simulink model "lib_nrhdlSignalDetection"  (R2023b)
settings: Solver=FixedStepDiscrete  StartTime=0.0  StopTime=sl_in.stopTime  RelTol=1e-3
undefined symbols (not defined in the file): sl_in
libraries: hdlsllib x5, simulink x4, dsphdlfiltering2 x4, dspsrcs4 x3, whdlmod x1
settings Model: DataTypeOverride=Off  SimulationMode=accelerator  Creator=The MathWorks, Inc.  LastModifiedBy=The MathWorks, Inc.
settings OptimizationCC: BlockReduction=off  ConditionallyExecuteInputs=off  DefaultParameterBehavior=Inlined  InheritOutputTypeSmallerThanSingle=on  ReuseModelBlockBuffer=off
settings DebuggingCC: AlgebraicLoopMsg=error  SingleTaskRateTransMsg=error  SubsystemReferenceDiagnosticForUnitTest=warning
settings HardwareCC: ProdBitPerPointer=32  ProdBitPerSizeT=32  ProdBitPerPtrDiffT=32  ProdLargestAtomicFloat=None  ProdIntDivRoundTo=Undefined  ProdEndianess=Unspecified  ProdWordSize=32  ProdHWDeviceType=ASIC/FPGA->ASIC/FPGA  TargetBitPerLong=64  TargetBitPerPointer=64  TargetBitPerSizeT=64  TargetBitPerPtrDiffT=64  TargetLongLongMode=on  TargetIntDivRoundTo=Zero  TargetEndianess=LittleEndian  TargetWordSize=64  TargetHWDeviceType=Custom Processor->MATLAB Host Computer  ProdEqTarget=off

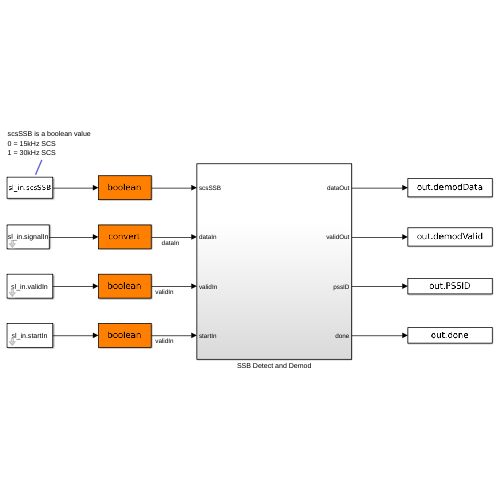
[thumbnail: Simulink's stored preview of the top-level diagram]
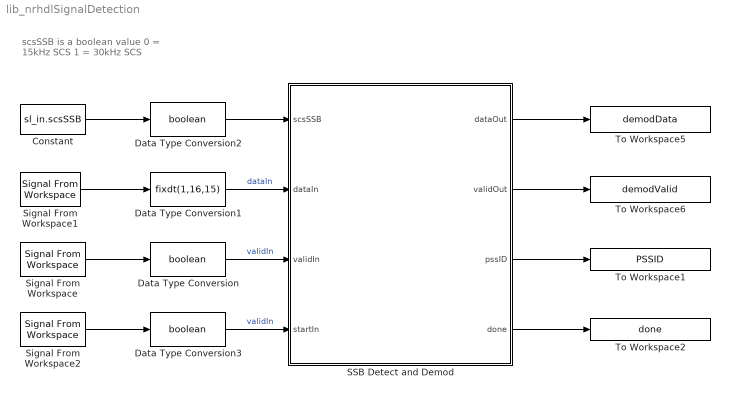
== system lib_nrhdlSignalDetection ==
  note: scsSSB is a boolean value
      | 0 = 15kHz SCS
      | 1 = 30kHz SCS
  Constant : Constant  Value=sl_in.scsSSB  SampleTime=sl_in.sampleTime
  Data Type Conversion : DataTypeConversion  OutDataTypeStr=boolean  SaturateOnIntegerOverflow=off  RndMeth=Floor
  Data Type Conversion1 : DataTypeConversion  OutDataTypeStr=fixdt(1,16,15)  RndMeth=Round  SaturateOnIntegerOverflow=off
  Data Type Conversion2 : DataTypeConversion  OutDataTypeStr=boolean  SaturateOnIntegerOverflow=off  RndMeth=Floor
  Data Type Conversion3 : DataTypeConversion  OutDataTypeStr=boolean  SaturateOnIntegerOverflow=off  RndMeth=Floor
  SSB Detect and Demod : Subsystem
  Signal From Workspace : dspsrcs4/Signal From Workspace  X=sl_in.validIn  Ts=sl_in.sampleTime  nsamps=1  OutputAfterFinalValue=Setting to zero  ignoreOrWarnInputAndFrameLengths=off  OutputFrames=off
  Signal From Workspace1 : dspsrcs4/Signal From Workspace  X=sl_in.signalIn  Ts=sl_in.sampleTime  nsamps=1  OutputAfterFinalValue=Setting to zero  ignoreOrWarnInputAndFrameLengths=off  OutputFrames=off
  Signal From Workspace2 : dspsrcs4/Signal From Workspace  X=sl_in.startIn  Ts=sl_in.sampleTime  nsamps=1  OutputAfterFinalValue=Setting to zero  ignoreOrWarnInputAndFrameLengths=off  OutputFrames=off
  To Workspace1 : ToWorkspace  VariableName=PSSID  SampleTime=-1
      settings: Save2DSignal=2-D array (concatenate along first dimension)
  To Workspace2 : ToWorkspace  VariableName=done  SampleTime=-1
      settings: Save2DSignal=2-D array (concatenate along first dimension)
  To Workspace5 : ToWorkspace  VariableName=demodData  SampleTime=-1
      settings: Save2DSignal=2-D array (concatenate along first dimension)
  To Workspace6 : ToWorkspace  VariableName=demodValid  SampleTime=-1
      settings: Save2DSignal=2-D array (concatenate along first dimension)
  wires:
  Signal From Workspace1/1 -> Data Type Conversion1/1
  Signal From Workspace/1 -> Data Type Conversion/1
  Data Type Conversion/1 -> SSB Detect and Demod/3(validIn)  "validIn"
  SSB Detect and Demod/1(dataOut) -> To Workspace5/1
  SSB Detect and Demod/2(validOut) -> To Workspace6/1
  Data Type Conversion1/1 -> SSB Detect and Demod/2(dataIn)  "dataIn"
  Constant/1 -> Data Type Conversion2/1
  SSB Detect and Demod/3(pssID) -> To Workspace1/1
  Data Type Conversion2/1 -> SSB Detect and Demod/1(scsSSB)
  Signal From Workspace2/1 -> Data Type Conversion3/1
  Data Type Conversion3/1 -> SSB Detect and Demod/4(startIn)  "validIn"
  SSB Detect and Demod/4(done) -> To Workspace2/1

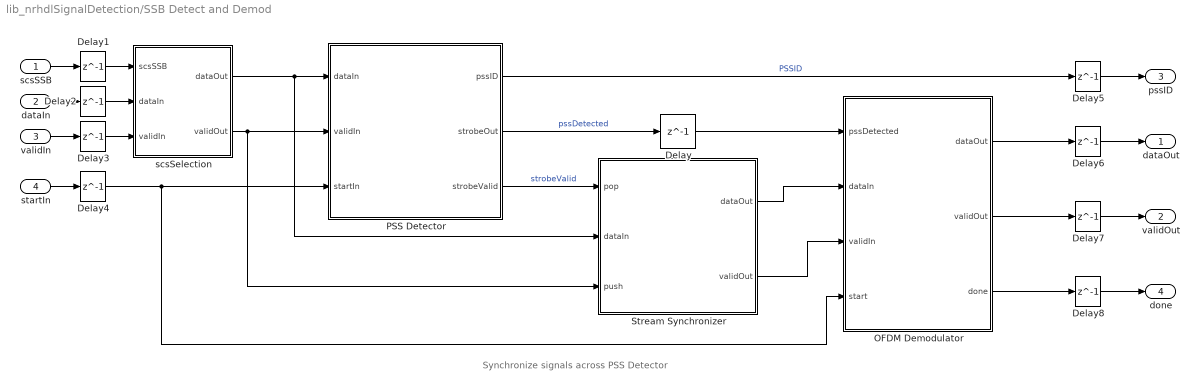
== system lib_nrhdlSignalDetection/SSB Detect and Demod ==
  note: Synchronize signals across PSS Detector
  scsSSB : Inport
  dataIn : Inport  Port=2
  validIn : Inport  Port=3
  startIn : Inport  Port=4
  Delay{,1..8} (9 alike) : Delay  DelayLength=1
  OFDM Demodulator : Subsystem
  PSS Detector : Subsystem
  Stream Synchronizer : Subsystem  mask{depth=512}
  scsSelection : Subsystem
  dataOut : Outport
  validOut : Outport  Port=2
  pssID : Outport  Port=3
  done : Outport  Port=4
  wires:
  OFDM Demodulator/1(dataOut) -> Delay6/1
  OFDM Demodulator/2(validOut) -> Delay7/1
  Stream Synchronizer/1(dataOut) -> OFDM Demodulator/2(dataIn)
  Stream Synchronizer/2(validOut) -> OFDM Demodulator/3(validIn)
  scsSelection/2(validOut) -> Stream Synchronizer/3(push), PSS Detector/2(validIn)
  PSS Detector/3(strobeValid) -> Stream Synchronizer/1(pop)  "strobeValid"
  scsSelection/1(dataOut) -> Stream Synchronizer/2(dataIn), PSS Detector/1(dataIn)
  PSS Detector/1(pssID) -> Delay5/1  "PSSID"
  scsSSB/1 -> Delay1/1
  validIn/1 -> Delay3/1
  dataIn/1 -> Delay2/1
  PSS Detector/2(strobeOut) -> Delay/1  "pssDetected"
  Delay/1 -> OFDM Demodulator/1(pssDetected)
  OFDM Demodulator/3(done) -> Delay8/1
  startIn/1 -> Delay4/1
  Delay1/1 -> scsSelection/1(scsSSB)
  Delay2/1 -> scsSelection/2(dataIn)
  Delay3/1 -> scsSelection/3(validIn)
  Delay4/1 -> OFDM Demodulator/4(start), PSS Detector/3(startIn)
  Delay5/1 -> pssID/1
  Delay6/1 -> dataOut/1
  Delay7/1 -> validOut/1
  Delay8/1 -> done/1

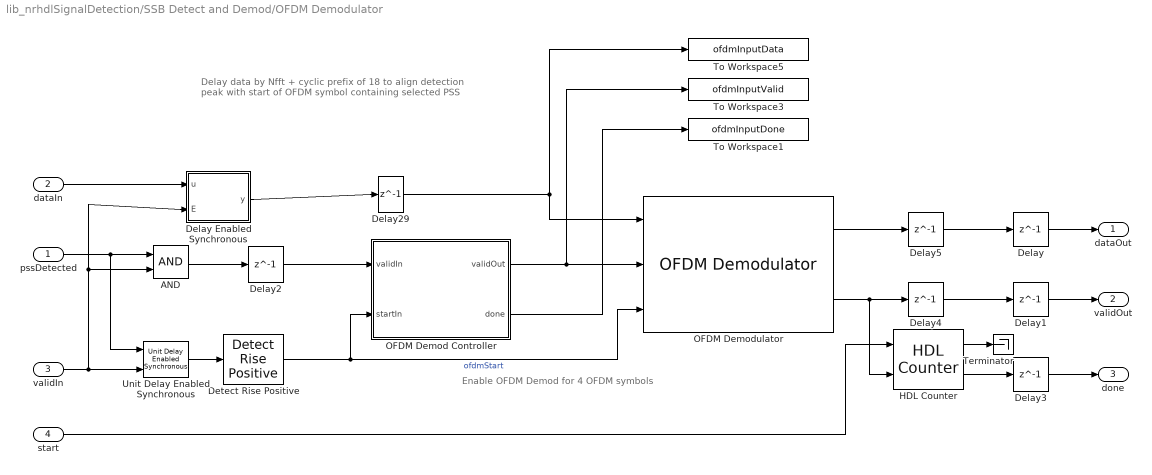
== system lib_nrhdlSignalDetection/SSB Detect and Demod/OFDM Demodulator ==
  note: Delay data by Nfft + cyclic prefix of 18 to align detection peak with start of OFDM symbol containing selected PSS
  note: Enable OFDM Demod for 4 OFDM symbols
  pssDetected : Inport
  dataIn : Inport  Port=2
  validIn : Inport  Port=3
  start : Inport  Port=4
  AND : Logic  AllPortsSameDT=off  OutDataTypeStr=boolean
  Delay{,1..5,29} (7 alike) : Delay  DelayLength=1
  Delay Enabled Synchronous : Subsystem  mask(Delay Enabled){DelayLength=256+18, InitialCondition=0.0}
      mask prompts: DelayLength "Simulink:blkprm_prompts:DelayBlkDelayLength"; InitialCondition "Simulink:blkprm_prompts:DelayBlkInitCond"
      mask help: Implements a delay with synchronous enable.
      mask TypeOptions DelayLength: Synchronous Delay/Delay/DelayLength
      mask TypeOptions InitialCondition: Synchronous Delay/Delay/InitialCondition
      mask DialogControl DelayLength Prompt: Delay length:
      mask DialogControl InitialCondition Prompt: Initial condition:
      mask Display:
      | port_label('input', 1, 'u');
      | port_label('input', 2, 'E');
      | text(0.45,0.45, 'Z');
      | DelayLengthStr = get_param(gcbh,'DelayLength');
      | try
      |     DelayLength = eval(DelayLengthStr);
      |     text(0.55,0.55, sprintf('-%d',DelayLength));
      | catch ME
      |     text(0.55,0.55, '-N');
      | end
  Detect Rise Positive : simulink/Logic and Bit Operations/Detect Rise Positive  vinit=0  OutDataTypeStr=boolean
  HDL Counter : hdlsllib/Sources/HDL Counter  CountType=Count limited  CountInit=0  CountStep=1  CountMax=960  CountFromType=Initial value  CountFrom=0  CountResetPort=on  CountLoadPort=off  CountEnbPort=on  CountDirPort=off  CountHitOutputPort=on  CountDataType=Unsigned  CountWordLen=12  CountFracLen=0  CountSampTime=1
  OFDM Demod Controller : MATLAB Function  TreatAsAtomicUnit=on
  OFDM Demodulator : whdlmod/OFDM Demodulator  OFDMParamsSource=Property  MaxFFTLength=256  FFTLength=256  CPLength=18  NumLGsC=8  NumRGsC=8  CPFraction=on  CPFractionSource=Property  CPFractionValue=0.5  removeDCSubcarriers=off  enableResetInputPort=on  Normalize=off  RoundingMethod=Round  SimulateUsing=Code generation
  Terminator : Terminator
  To Workspace1 : ToWorkspace  VariableName=ofdmInputDone  SampleTime=-1
      settings: Save2DSignal=2-D array (concatenate along first dimension)
  To Workspace3 : ToWorkspace  VariableName=ofdmInputValid  SampleTime=-1
      settings: Save2DSignal=2-D array (concatenate along first dimension)
  To Workspace5 : ToWorkspace  VariableName=ofdmInputData  SampleTime=-1
      settings: Save2DSignal=2-D array (concatenate along first dimension)
  Unit Delay Enabled Synchronous : hdlsllib/Discrete/Unit Delay Enabled Synchronous  InitialCondition=0.0  SampleTime=-1
  dataOut : Outport
  validOut : Outport  Port=2
  done : Outport  Port=3
  wires:
  AND/1 -> Delay2/1
  pssDetected/1 -> Unit Delay Enabled Synchronous/1, AND/1
  Unit Delay Enabled Synchronous/1 -> Detect Rise Positive/1
  dataIn/1 -> Delay Enabled Synchronous/1(u)
  Delay Enabled Synchronous/1(y) -> Delay29/1
  Delay29/1 -> OFDM Demodulator/1, To Workspace5/1
  Delay2/1 -> OFDM Demod Controller/1(validIn)
  Detect Rise Positive/1 -> OFDM Demodulator/3, OFDM Demod Controller/2(startIn)  "ofdmStart"
  OFDM Demod Controller/1(validOut) -> OFDM Demodulator/2, To Workspace3/1
  OFDM Demod Controller/2(done) -> To Workspace1/1
  HDL Counter/2 -> Delay3/1
  validIn/1 -> Delay Enabled Synchronous/2(E), AND/2, Unit Delay Enabled Synchronous/2
  HDL Counter/1 -> Terminator/1
  Delay/1 -> dataOut/1
  Delay1/1 -> validOut/1
  Delay3/1 -> done/1
  start/1 -> HDL Counter/1
  OFDM Demodulator/2 -> Delay4/1, HDL Counter/2
  OFDM Demodulator/1 -> Delay5/1
  Delay5/1 -> Delay/1
  Delay4/1 -> Delay1/1

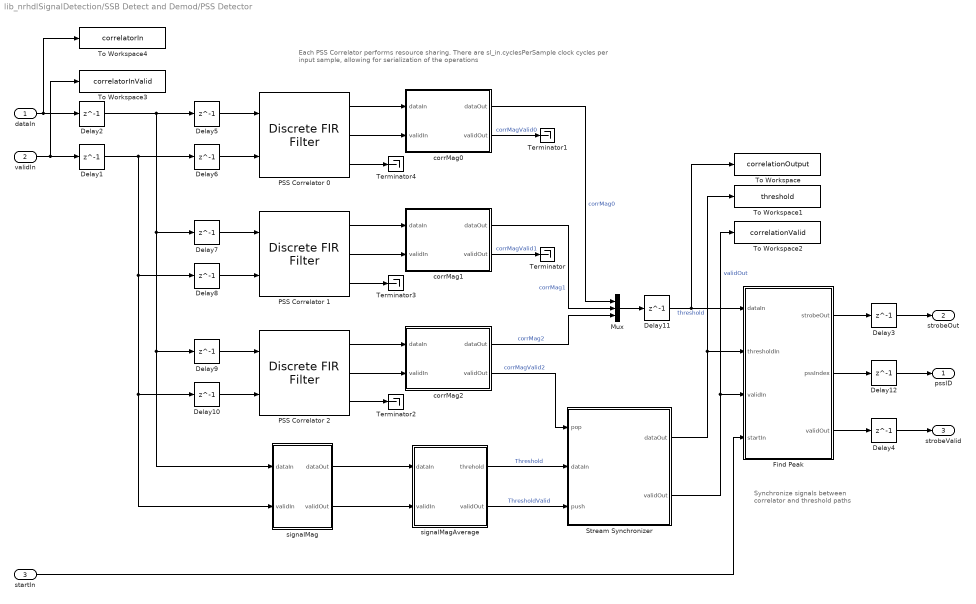
== system lib_nrhdlSignalDetection/SSB Detect and Demod/PSS Detector ==
  note: Each PSS Correlator performs resource sharing. There are sl_in.cyclesPerSample clock cycles per input sample, allowing for serialization of the operations
  note: Synchronize signals between correlator and threshold paths
  dataIn : Inport
  validIn : Inport  Port=2
  startIn : Inport  Port=3
  Delay{1..12} (12 alike) : Delay  DelayLength=1
  Find Peak : Subsystem
  Mux : Mux  Inputs=3
  PSS Correlator 0 : dsphdlfiltering2/Discrete FIR Filter  NumeratorSource=Property  Numerator=sl_in.pssCorrelationCoeffs(:,1).'  NumeratorPrototype=[]  FilterStructure=Partly serial systolic  SerializationOption=Minimum number of cycles between valid input samples  NumCycles=sl_in.cyclesPerSample  NumberOfMultipliers=2  SimulateUsing=Code generation  roundingMode=Floor  overflowMode=off  CoefficientsDataTypeStr=fixdt(1,8,10)  OutputDataTypeStr=fixdt(1,18,13)  ResetInputPort=off  HDLGlobalReset=off  CoeffMultiplier=Multiplier  UseMultForPow2Coeff=on
  PSS Correlator 1 : dsphdlfiltering2/Discrete FIR Filter  NumeratorSource=Property  Numerator=sl_in.pssCorrelationCoeffs(:,2).'  NumeratorPrototype=[]  FilterStructure=Partly serial systolic  SerializationOption=Minimum number of cycles between valid input samples  NumCycles=sl_in.cyclesPerSample  NumberOfMultipliers=2  SimulateUsing=Code generation  roundingMode=Floor  overflowMode=off  CoefficientsDataTypeStr=fixdt(1,8,10)  OutputDataTypeStr=fixdt(1,18,13)  ResetInputPort=off  HDLGlobalReset=off  CoeffMultiplier=Multiplier  UseMultForPow2Coeff=on
  PSS Correlator 2 : dsphdlfiltering2/Discrete FIR Filter  NumeratorSource=Property  Numerator=sl_in.pssCorrelationCoeffs(:,3).'  NumeratorPrototype=[]  FilterStructure=Partly serial systolic  SerializationOption=Minimum number of cycles between valid input samples  NumCycles=sl_in.cyclesPerSample  NumberOfMultipliers=2  SimulateUsing=Code generation  roundingMode=Floor  overflowMode=off  CoefficientsDataTypeStr=fixdt(1,8,10)  OutputDataTypeStr=fixdt(1,18,13)  ResetInputPort=off  HDLGlobalReset=off  CoeffMultiplier=Multiplier  UseMultForPow2Coeff=on
  Stream Synchronizer : Subsystem  mask{depth=512}
  Terminator{,1..4} (5 alike) : Terminator
  To Workspace : ToWorkspace  VariableName=correlationOutput  SampleTime=-1
      settings: Save2DSignal=2-D array (concatenate along first dimension)
  To Workspace1 : ToWorkspace  VariableName=threshold  SampleTime=-1
      settings: Save2DSignal=2-D array (concatenate along first dimension)
  To Workspace2 : ToWorkspace  VariableName=correlationValid  SampleTime=-1
      settings: Save2DSignal=2-D array (concatenate along first dimension)
  To Workspace3 : ToWorkspace  VariableName=correlatorInValid  SampleTime=-1
      settings: Save2DSignal=2-D array (concatenate along first dimension)
  To Workspace4 : ToWorkspace  VariableName=correlatorIn  SampleTime=-1
      settings: Save2DSignal=2-D array (concatenate along first dimension)
  corrMag0 : Subsystem
  corrMag1 : Subsystem
  corrMag2 : Subsystem
  signalMag : Subsystem
  signalMagAverage : Subsystem
  pssID : Outport
  strobeOut : Outport  Port=2
  strobeValid : Outport  Port=3
  wires:
  Stream Synchronizer/2(validOut) -> To Workspace2/1, Find Peak/3(validIn)  "validOut"
  Stream Synchronizer/1(dataOut) -> To Workspace1/1, Find Peak/2(thresholdIn)  "threshold"
  signalMagAverage/2(validOut) -> Stream Synchronizer/3(push)  "ThresholdValid"
  signalMagAverage/1(threhold) -> Stream Synchronizer/2(dataIn)  "Threshold"
  signalMag/2(validOut) -> signalMagAverage/2(validIn)
  signalMag/1(dataOut) -> signalMagAverage/1(dataIn)
  Delay4/1 -> strobeValid/1
  Find Peak/1(strobeOut) -> Delay3/1
  corrMag2/2(validOut) -> Stream Synchronizer/1(pop)  "corrMagValid2"
  Find Peak/3(validOut) -> Delay4/1
  validIn/1 -> To Workspace3/1, Delay1/1
  PSS Correlator 2/1 -> corrMag2/1(dataIn)
  PSS Correlator 2/2 -> corrMag2/2(validIn)
  dataIn/1 -> To Workspace4/1, Delay2/1
  PSS Correlator 1/2 -> corrMag1/2(validIn)
  PSS Correlator 1/1 -> corrMag1/1(dataIn)
  PSS Correlator 0/1 -> corrMag0/1(dataIn)
  PSS Correlator 0/2 -> corrMag0/2(validIn)
  corrMag1/2(validOut) -> Terminator/1  "corrMagValid1"
  corrMag0/2(validOut) -> Terminator1/1  "corrMagValid0"
  Delay5/1 -> PSS Correlator 0/1
  Delay6/1 -> PSS Correlator 0/2
  Delay8/1 -> PSS Correlator 1/2
  Delay7/1 -> PSS Correlator 1/1
  Delay9/1 -> PSS Correlator 2/1
  Delay1/1 -> signalMag/2(validIn), Delay10/1, Delay8/1, Delay6/1
  Delay10/1 -> PSS Correlator 2/2
  Delay2/1 -> Delay9/1, signalMag/1(dataIn), Delay7/1, Delay5/1
  PSS Correlator 2/3 -> Terminator2/1
  PSS Correlator 1/3 -> Terminator3/1
  PSS Correlator 0/3 -> Terminator4/1
  corrMag0/1(dataOut) -> Mux/1  "corrMag0"
  corrMag1/1(dataOut) -> Mux/2  "corrMag1"
  corrMag2/1(dataOut) -> Mux/3  "corrMag2"
  Delay3/1 -> strobeOut/1
  Find Peak/2(pssIndex) -> Delay12/1
  Delay12/1 -> pssID/1
  Mux/1 -> Delay11/1
  Delay11/1 -> To Workspace/1, Find Peak/1(dataIn)
  startIn/1 -> Find Peak/4(startIn)

== system lib_nrhdlSignalDetection/SSB Detect and Demod/Stream Synchronizer ==
  pop : Inport
  dataIn : Inport  Port=2
  push : Inport  Port=3
  MATLAB Function : MATLAB Function  InitFcn=Simulink.suppressDiagnostic(gcb, 'Stateflow:Runtime:DataOverflowErrorMSLD');  TreatAsAtomicUnit=on
  Simple Dual Port RAM System : hdlsllib/HDL RAMs/Simple Dual Port RAM System  RAMType=Simple dual port  AsyncRead=off  WriteOutputValue=New data  RAMInitialValue=0  allowBusInputs=off  WritesHaveOutput=on  NumReads=0  NumWrites=1  SimulateUsing=Code generation
  dataOut : Outport
  validOut : Outport  Port=2
  wires:
  Simple Dual Port RAM System/1 -> dataOut/1
  dataIn/1 -> Simple Dual Port RAM System/1
  pop/1 -> MATLAB Function/1(pop)
  push/1 -> MATLAB Function/2(push)
  MATLAB Function/4(validOut) -> validOut/1
  MATLAB Function/1(wrAddr) -> Simple Dual Port RAM System/2
  MATLAB Function/2(wrEn) -> Simple Dual Port RAM System/3
  MATLAB Function/3(rdAddr) -> Simple Dual Port RAM System/4

== system lib_nrhdlSignalDetection/SSB Detect and Demod/scsSelection ==
  note: 0 = 15kHz SCS
      | 1 = 30kHz SCS
  note: Decimate to 15KHz SCS rate
  note: convert to sfix16_15 to match filter input data type
  scsSSB : Inport
  dataIn : Inport  Port=2
  validIn : Inport  Port=3
  Data Type Conversion : DataTypeConversion  OutDataTypeStr=fixdt(1,16,15)  RndMeth=Round  SaturateOnIntegerOverflow=off
  FIR Decimator : dsphdlfiltering2/FIR Decimator  Numerator=sl_in.halfbandCoeffs  FilterStructure=Direct form systolic  DecimationFactor=2  NumCycles=sl_in.cyclesPerSample  SimulateUsing=Code generation  roundingMode=Round  overflowMode=off  CoefficientsDataTypeStr=fixdt(1,16,16)  ResetInputPort=off  HDLGlobalReset=off
  Multiport Switch : MultiPortSwitch  DataPortOrder=Zero-based contiguous  Inputs=2  zeroidx=on  SaturateOnIntegerOverflow=off  InputSameDT=off
  Multiport Switch1 : MultiPortSwitch  DataPortOrder=Zero-based contiguous  Inputs=2  zeroidx=on  SaturateOnIntegerOverflow=off  InputSameDT=off
  Transient Removal : MATLAB Function  TreatAsAtomicUnit=on  mask{TransientLength=sl_in.halfbandTransient}
      mask prompts: TransientLength "Transient length"
  dataOut : Outport
  validOut : Outport  Port=2
  wires:
  Multiport Switch/1 -> dataOut/1
  Multiport Switch1/1 -> validOut/1
  scsSSB/1 -> Multiport Switch1/1, Multiport Switch/1
  FIR Decimator/1 -> Data Type Conversion/1
  dataIn/1 -> Multiport Switch/3, FIR Decimator/1
  validIn/1 -> Multiport Switch1/3, FIR Decimator/2
  FIR Decimator/2 -> Transient Removal/2(validIn)
  Data Type Conversion/1 -> Transient Removal/1(dataIn)
  Transient Removal/1(dataOut) -> Multiport Switch/2
  Transient Removal/2(validOut) -> Multiport Switch1/2

== system lib_nrhdlSignalDetection/SSB Detect and Demod/OFDM Demodulator/Delay Enabled Synchronous ==
  u : Inport
  E : Inport  Port=2
  Synchronous Delay : Subsystem
  y : Outport
  wires:
  Synchronous Delay/1(y) -> y/1
  E/1 -> Synchronous Delay/2(E)
  u/1 -> Synchronous Delay/1(u)

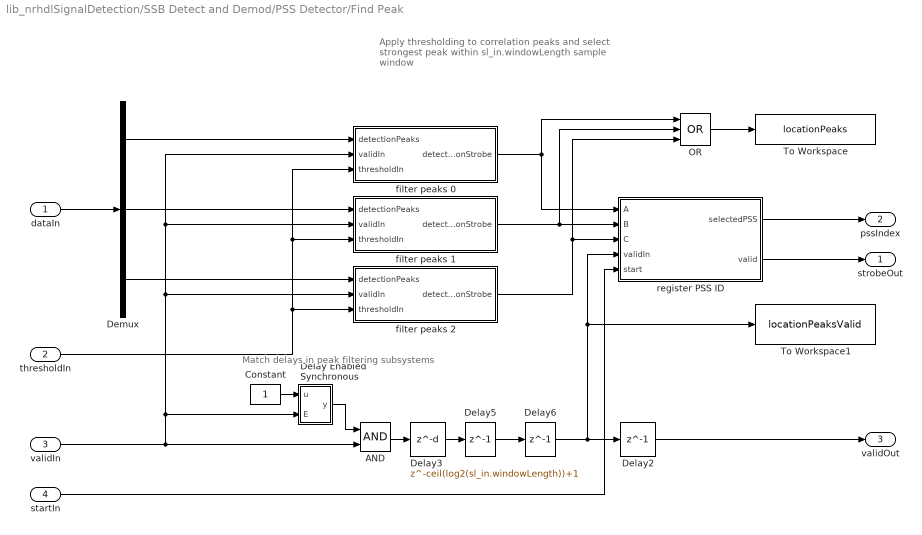
== system lib_nrhdlSignalDetection/SSB Detect and Demod/PSS Detector/Find Peak ==
  note: Match delays in peak filtering subsystems
  note: Apply thresholding to correlation peaks and select strongest peak within sl_in.windowLength sample window
  dataIn : Inport
  thresholdIn : Inport  Port=2
  validIn : Inport  Port=3
  startIn : Inport  Port=4
  AND : Logic  AllPortsSameDT=off  OutDataTypeStr=boolean
  Constant : Constant  OutDataTypeStr=boolean  SampleTime=-1
  Delay Enabled Synchronous : Subsystem  mask(Delay Enabled){DelayLength=ceil(sl_in.windowLength/2), InitialCondition=0.0}
      mask prompts: DelayLength "Simulink:blkprm_prompts:DelayBlkDelayLength"; InitialCondition "Simulink:blkprm_prompts:DelayBlkInitCond"
      mask help: Implements a delay with synchronous enable.
      mask TypeOptions DelayLength: Synchronous Delay/Delay/DelayLength
      mask TypeOptions InitialCondition: Synchronous Delay/Delay/InitialCondition
      mask DialogControl DelayLength Prompt: Delay length:
      mask DialogControl InitialCondition Prompt: Initial condition:
      mask Display:
      | port_label('input', 1, 'u');
      | port_label('input', 2, 'E');
      | text(0.45,0.45, 'Z');
      | DelayLengthStr = get_param(gcbh,'DelayLength');
      | try
      |     DelayLength = eval(DelayLengthStr);
      |     text(0.55,0.55, sprintf('-%d',DelayLength));
      | catch ME
      |     text(0.55,0.55, '-N');
      | end
  Delay2 : Delay  DelayLength=1
  Delay3 : Delay  DelayLength=ceil(log2(sl_in.windowLength))+1
  Delay5 : Delay  DelayLength=1
  Delay6 : Delay  DelayLength=1
  Demux : Demux  Outputs=3
  OR : Logic  Operator=OR  Inputs=3  AllPortsSameDT=off  OutDataTypeStr=boolean
  To Workspace : ToWorkspace  VariableName=locationPeaks  SampleTime=-1
      settings: Save2DSignal=2-D array (concatenate along first dimension)
  To Workspace1 : ToWorkspace  VariableName=locationPeaksValid  SampleTime=-1
      settings: Save2DSignal=2-D array (concatenate along first dimension)
  filter peaks 0 : Subsystem
  filter peaks 1 : Subsystem
  filter peaks 2 : Subsystem
  register PSS ID : MATLAB Function  TreatAsAtomicUnit=on
  strobeOut : Outport
  pssIndex : Outport  Port=2
  validOut : Outport  Port=3
  wires:
  Delay6/1 -> register PSS ID/4(validIn), To Workspace1/1, Delay2/1
  Delay5/1 -> Delay6/1
  validIn/1 -> AND/2, filter peaks 2/2(validIn), filter peaks 1/2(validIn), filter peaks 0/2(validIn), Delay Enabled Synchronous/2(E)
  dataIn/1 -> Demux/1
  register PSS ID/1(selectedPSS) -> pssIndex/1
  Demux/2 -> filter peaks 1/1(detectionPeaks)
  Demux/3 -> filter peaks 2/1(detectionPeaks)
  thresholdIn/1 -> filter peaks 2/3(thresholdIn), filter peaks 1/3(thresholdIn), filter peaks 0/3(thresholdIn)
  Demux/1 -> filter peaks 0/1(detectionPeaks)
  filter peaks 0/1(detectionStrobe) -> OR/1, register PSS ID/1(A)
  filter peaks 1/1(detectionStrobe) -> OR/2, register PSS ID/2(B)
  filter peaks 2/1(detectionStrobe) -> OR/3, register PSS ID/3(C)
  register PSS ID/2(valid) -> strobeOut/1
  Delay2/1 -> validOut/1
  OR/1 -> To Workspace/1
  Delay Enabled Synchronous/1(y) -> AND/1
  Constant/1 -> Delay Enabled Synchronous/1(u)
  AND/1 -> Delay3/1
  startIn/1 -> register PSS ID/5(start)
  Delay3/1 -> Delay5/1

== system lib_nrhdlSignalDetection/SSB Detect and Demod/PSS Detector/Stream Synchronizer ==
  pop : Inport
  dataIn : Inport  Port=2
  push : Inport  Port=3
  MATLAB Function : MATLAB Function  InitFcn=Simulink.suppressDiagnostic(gcb, 'Stateflow:Runtime:DataOverflowErrorMSLD');  TreatAsAtomicUnit=on
  Simple Dual Port RAM System : hdlsllib/HDL RAMs/Simple Dual Port RAM System  RAMType=Simple dual port  AsyncRead=off  WriteOutputValue=New data  RAMInitialValue=0  allowBusInputs=off  WritesHaveOutput=on  NumReads=0  NumWrites=1  SimulateUsing=Code generation
  dataOut : Outport
  validOut : Outport  Port=2
  wires:
  Simple Dual Port RAM System/1 -> dataOut/1
  dataIn/1 -> Simple Dual Port RAM System/1
  pop/1 -> MATLAB Function/1(pop)
  push/1 -> MATLAB Function/2(push)
  MATLAB Function/4(validOut) -> validOut/1
  MATLAB Function/1(wrAddr) -> Simple Dual Port RAM System/2
  MATLAB Function/2(wrEn) -> Simple Dual Port RAM System/3
  MATLAB Function/3(rdAddr) -> Simple Dual Port RAM System/4

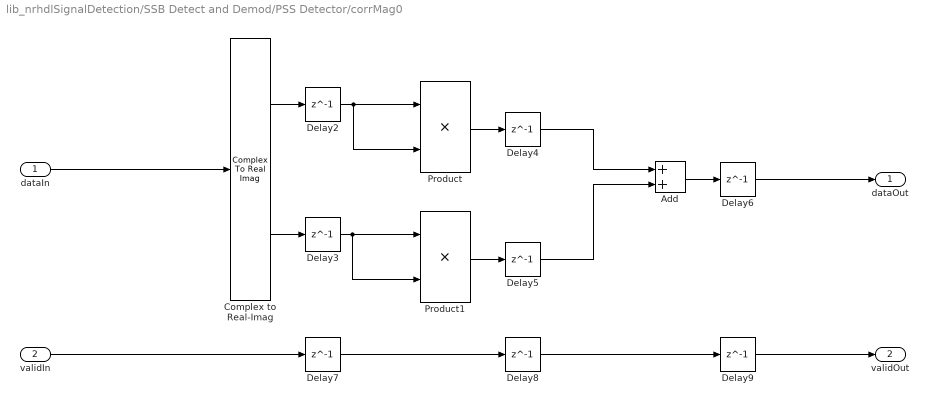
== system lib_nrhdlSignalDetection/SSB Detect and Demod/PSS Detector/corrMag0 ==
  dataIn : Inport
  validIn : Inport  Port=2
  Add : Sum  OutDataTypeStr=Inherit: Same as accumulator
  Complex to Real-Imag : ComplexToRealImag
  Delay{2..9} (8 alike) : Delay  DelayLength=1
  Product : Product
  Product1 : Product
  dataOut : Outport
  validOut : Outport  Port=2
  wires:
  validIn/1 -> Delay7/1
  dataIn/1 -> Complex to Real-Imag/1
  Product/1 -> Delay4/1
  Delay3/1 -> Product1/1, Product1/2
  Delay7/1 -> Delay8/1
  Delay5/1 -> Add/2
  Delay6/1 -> dataOut/1
  Product1/1 -> Delay5/1
  Delay9/1 -> validOut/1
  Delay4/1 -> Add/1
  Complex to Real-Imag/2 -> Delay3/1
  Delay8/1 -> Delay9/1
  Complex to Real-Imag/1 -> Delay2/1
  Add/1 -> Delay6/1
  Delay2/1 -> Product/1, Product/2

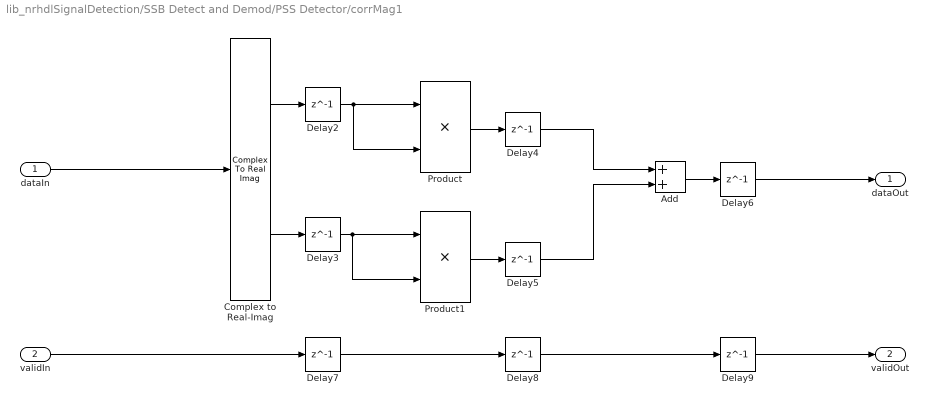
== system lib_nrhdlSignalDetection/SSB Detect and Demod/PSS Detector/corrMag1 ==
  dataIn : Inport
  validIn : Inport  Port=2
  Add : Sum  OutDataTypeStr=Inherit: Same as accumulator
  Complex to Real-Imag : ComplexToRealImag
  Delay{2..9} (8 alike) : Delay  DelayLength=1
  Product : Product
  Product1 : Product
  dataOut : Outport
  validOut : Outport  Port=2
  wires:
  Delay2/1 -> Product/2, Product/1
  Add/1 -> Delay6/1
  Complex to Real-Imag/1 -> Delay2/1
  Delay8/1 -> Delay9/1
  Complex to Real-Imag/2 -> Delay3/1
  Delay4/1 -> Add/1
  Delay9/1 -> validOut/1
  Product1/1 -> Delay5/1
  Delay6/1 -> dataOut/1
  Delay5/1 -> Add/2
  Delay7/1 -> Delay8/1
  Delay3/1 -> Product1/2, Product1/1
  Product/1 -> Delay4/1
  dataIn/1 -> Complex to Real-Imag/1
  validIn/1 -> Delay7/1

== system lib_nrhdlSignalDetection/SSB Detect and Demod/PSS Detector/corrMag2 ==
  dataIn : Inport
  validIn : Inport  Port=2
  Add : Sum  OutDataTypeStr=Inherit: Same as accumulator
  Complex to Real-Imag : ComplexToRealImag
  Delay{2..9} (8 alike) : Delay  DelayLength=1
  Product : Product
  Product1 : Product
  dataOut : Outport
  validOut : Outport  Port=2
  wires:
  validIn/1 -> Delay7/1
  dataIn/1 -> Complex to Real-Imag/1
  Product/1 -> Delay4/1
  Delay3/1 -> Product1/1, Product1/2
  Delay7/1 -> Delay8/1
  Delay5/1 -> Add/2
  Delay6/1 -> dataOut/1
  Product1/1 -> Delay5/1
  Delay9/1 -> validOut/1
  Delay4/1 -> Add/1
  Complex to Real-Imag/2 -> Delay3/1
  Delay8/1 -> Delay9/1
  Complex to Real-Imag/1 -> Delay2/1
  Add/1 -> Delay6/1
  Delay2/1 -> Product/1, Product/2

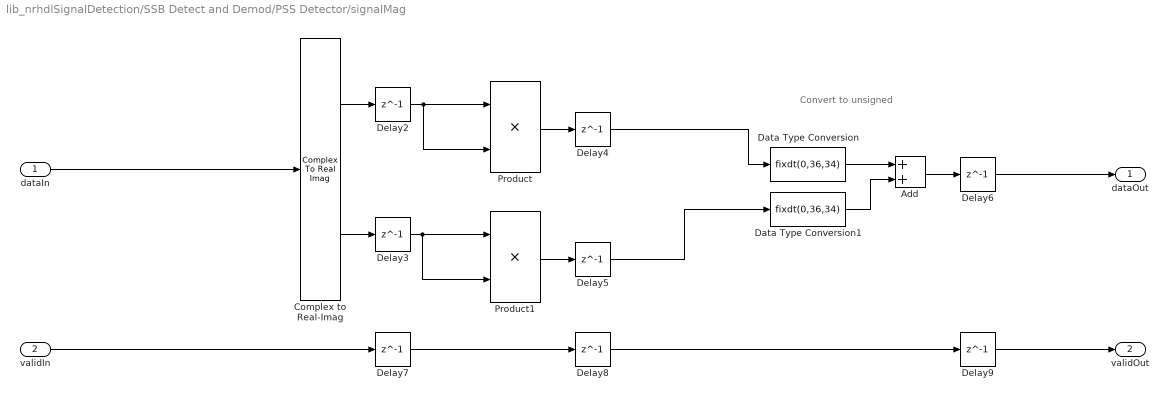
== system lib_nrhdlSignalDetection/SSB Detect and Demod/PSS Detector/signalMag ==
  note: Convert to unsigned
  dataIn : Inport
  validIn : Inport  Port=2
  Add : Sum
  Complex to Real-Imag : ComplexToRealImag
  Data Type Conversion : DataTypeConversion  OutDataTypeStr=fixdt(0,36,34)  SaturateOnIntegerOverflow=off  RndMeth=Floor
  Data Type Conversion1 : DataTypeConversion  OutDataTypeStr=fixdt(0,36,34)  SaturateOnIntegerOverflow=off  RndMeth=Floor
  Delay{2..9} (8 alike) : Delay  DelayLength=1
  Product : Product
  Product1 : Product
  dataOut : Outport
  validOut : Outport  Port=2
  wires:
  Data Type Conversion1/1 -> Add/2
  Data Type Conversion/1 -> Add/1
  Delay2/1 -> Product/2, Product/1
  Add/1 -> Delay6/1
  Complex to Real-Imag/1 -> Delay2/1
  Delay8/1 -> Delay9/1
  Complex to Real-Imag/2 -> Delay3/1
  Delay4/1 -> Data Type Conversion/1
  Delay9/1 -> validOut/1
  Product1/1 -> Delay5/1
  Delay6/1 -> dataOut/1
  Delay5/1 -> Data Type Conversion1/1
  Delay7/1 -> Delay8/1
  Delay3/1 -> Product1/2, Product1/1
  Product/1 -> Delay4/1
  dataIn/1 -> Complex to Real-Imag/1
  validIn/1 -> Delay7/1

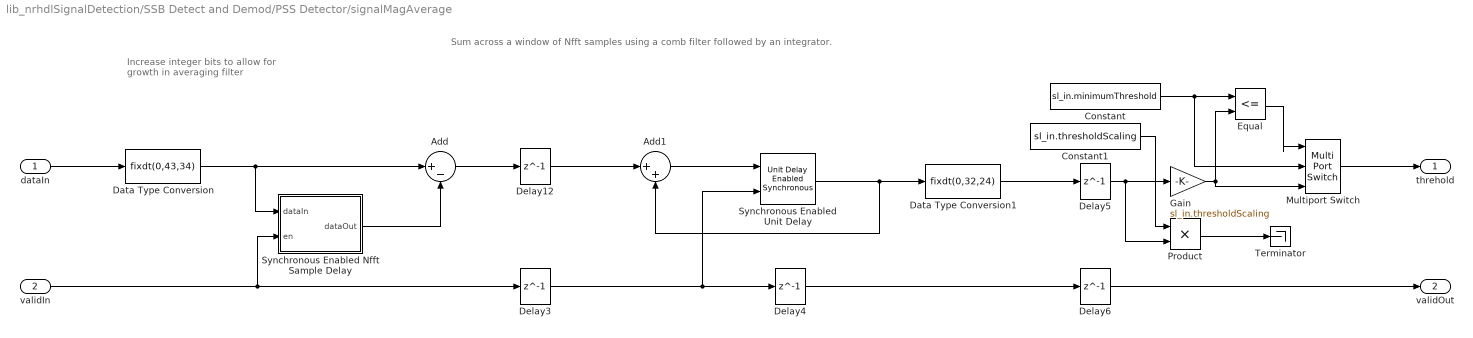
== system lib_nrhdlSignalDetection/SSB Detect and Demod/PSS Detector/signalMagAverage ==
  note: Increase integer bits to allow for growth in averaging filter
  note: Sum across a window of Nfft samples using a comb filter followed by an integrator.
  dataIn : Inport
  validIn : Inport  Port=2
  Add : Sum  Inputs=|+-  OutDataTypeStr=Inherit: Same as accumulator
  Add1 : Sum  Inputs=|++  OutDataTypeStr=Inherit: Same as accumulator
  Constant : Constant  Value=sl_in.minimumThreshold  SampleTime=-1
  Constant1 : Constant  Value=sl_in.thresholdScaling  SampleTime=-1
  Data Type Conversion : DataTypeConversion  OutDataTypeStr=fixdt(0,43,34)  SaturateOnIntegerOverflow=off  RndMeth=Floor
  Data Type Conversion1 : DataTypeConversion  OutDataTypeStr=fixdt(0,32,24)  SaturateOnIntegerOverflow=off  RndMeth=Floor
  Delay{3..6,12} (5 alike) : Delay  DelayLength=1  InitialCondition=0
  Equal : RelationalOperator  Operator=<=  OutDataTypeStr=boolean  RndMeth=Simplest  InputSameDT=off
  Gain : Gain  Gain=sl_in.thresholdScaling  ParamDataTypeStr=Inherit: Inherit from 'Gain'  OutDataTypeStr=Inherit: Same as input
  Multiport Switch : MultiPortSwitch  DataPortOrder=Zero-based contiguous  Inputs=2  zeroidx=on  SaturateOnIntegerOverflow=off  InputSameDT=off
  Product : Product
  "Synchronous Enabled Nfft Sample Delay " : Subsystem
  Synchronous Enabled Unit Delay : hdlsllib/Discrete/Unit Delay Enabled Synchronous  InitialCondition=0.0  SampleTime=-1
  Terminator : Terminator
  threhold : Outport  VectorParamsAs1DForOutWhenUnconnected=off
  validOut : Outport  Port=2  VectorParamsAs1DForOutWhenUnconnected=off
  wires:
  "Synchronous Enabled Nfft Sample Delay "/1(dataOut) -> Add/2
  Data Type Conversion1/1 -> Delay5/1
  Data Type Conversion/1 -> Add/1, "Synchronous Enabled Nfft Sample Delay "/1(dataIn)
  Delay6/1 -> validOut/1
  Delay5/1 -> Product/2, Gain/1
  Delay4/1 -> Delay6/1
  Delay3/1 -> Delay4/1, Synchronous Enabled Unit Delay/2
  Delay12/1 -> Add1/1
  validIn/1 -> Delay3/1, "Synchronous Enabled Nfft Sample Delay "/2(en)
  Add/1 -> Delay12/1
  Add1/1 -> Synchronous Enabled Unit Delay/1
  dataIn/1 -> Data Type Conversion/1
  Synchronous Enabled Unit Delay/1 -> Add1/2, Data Type Conversion1/1
  Equal/1 -> Multiport Switch/1
  Constant/1 -> Multiport Switch/2, Equal/1
  Gain/1 -> Equal/2, Multiport Switch/3
  Multiport Switch/1 -> threhold/1
  Constant1/1 -> Product/1
  Product/1 -> Terminator/1

== system lib_nrhdlSignalDetection/SSB Detect and Demod/OFDM Demodulator/Delay Enabled Synchronous/Synchronous Delay ==
  u : Inport
  E : Inport  Port=2
  Delay : Delay  DelayLength=DelayLength  InitialCondition=InitialCondition  ShowEnablePort=on
      settings: InputPortMap=u0,e6
  State Control : StateControl  StateControl=Synchronous
  y : Outport
  wires:
  u/1 -> Delay/1
  E/1 -> Delay/2
  Delay/1 -> y/1

== system lib_nrhdlSignalDetection/SSB Detect and Demod/PSS Detector/Find Peak/Delay Enabled Synchronous ==
  u : Inport
  E : Inport  Port=2
  Synchronous Delay : Subsystem
  y : Outport
  wires:
  Synchronous Delay/1(y) -> y/1
  E/1 -> Synchronous Delay/2(E)
  u/1 -> Synchronous Delay/1(u)

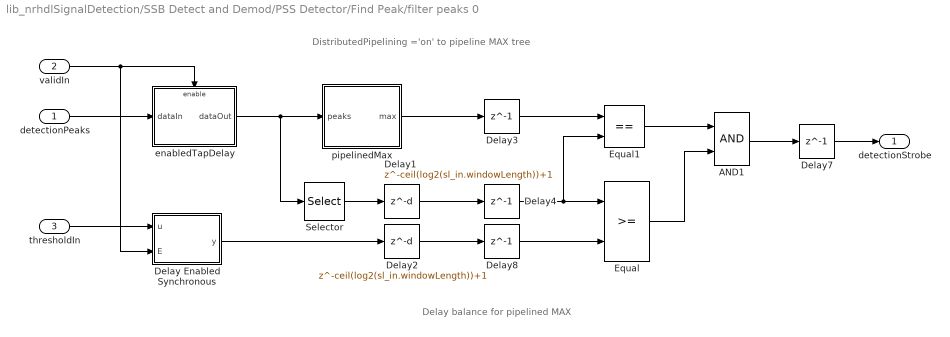
== system lib_nrhdlSignalDetection/SSB Detect and Demod/PSS Detector/Find Peak/filter peaks 0 ==
  note: Delay balance for pipelined MAX
  note: DistributedPipelining ='on' to pipeline MAX tree
  detectionPeaks : Inport
  validIn : Inport  Port=2
  thresholdIn : Inport  Port=3
  AND1 : Logic  AllPortsSameDT=off  OutDataTypeStr=boolean
  Delay Enabled Synchronous : Subsystem  mask(Delay Enabled){DelayLength=ceil(sl_in.windowLength/2), InitialCondition=0.0}
      mask prompts: DelayLength "Simulink:blkprm_prompts:DelayBlkDelayLength"; InitialCondition "Simulink:blkprm_prompts:DelayBlkInitCond"
      mask help: Implements a delay with synchronous enable.
      mask TypeOptions DelayLength: Synchronous Delay/Delay/DelayLength
      mask TypeOptions InitialCondition: Synchronous Delay/Delay/InitialCondition
      mask DialogControl DelayLength Prompt: Delay length:
      mask DialogControl InitialCondition Prompt: Initial condition:
      mask Display:
      | port_label('input', 1, 'u');
      | port_label('input', 2, 'E');
      | text(0.45,0.45, 'Z');
      | DelayLengthStr = get_param(gcbh,'DelayLength');
      | try
      |     DelayLength = eval(DelayLengthStr);
      |     text(0.55,0.55, sprintf('-%d',DelayLength));
      | catch ME
      |     text(0.55,0.55, '-N');
      | end
  Delay1 : Delay  DelayLength=ceil(log2(sl_in.windowLength))+1
  Delay2 : Delay  DelayLength=ceil(log2(sl_in.windowLength))+1
  Delay3 : Delay  DelayLength=1
  Delay4 : Delay  DelayLength=1
  Delay7 : Delay  DelayLength=1
  Delay8 : Delay  DelayLength=1  InitialCondition=1
  Equal : RelationalOperator  OutDataTypeStr=boolean  RndMeth=Simplest  InputSameDT=off
  Equal1 : RelationalOperator  Operator===  OutDataTypeStr=boolean  RndMeth=Simplest  InputSameDT=off
  Selector : Selector  InputPortWidth=sl_in.windowLength  IndexOptions=Index vector (dialog)  Indices=ceil(sl_in.windowLength/2)  OutputSizes=1
  enabledTapDelay : Subsystem
  pipelinedMax : Subsystem
  detectionStrobe : Outport
  wires:
  Equal1/1 -> AND1/1
  Delay4/1 -> Equal1/2, Equal/1
  Delay3/1 -> Equal1/1
  Equal/1 -> AND1/2
  AND1/1 -> Delay7/1
  Selector/1 -> Delay1/1
  Delay8/1 -> Equal/2
  Delay7/1 -> detectionStrobe/1
  thresholdIn/1 -> Delay Enabled Synchronous/1(u)
  validIn/1 -> Delay Enabled Synchronous/2(E), enabledTapDelay/Enable
  Delay Enabled Synchronous/1(y) -> Delay2/1
  enabledTapDelay/1(dataOut) -> Selector/1, pipelinedMax/1(peaks)
  detectionPeaks/1 -> enabledTapDelay/1(dataIn)
  pipelinedMax/1(max) -> Delay3/1
  Delay1/1 -> Delay4/1
  Delay2/1 -> Delay8/1

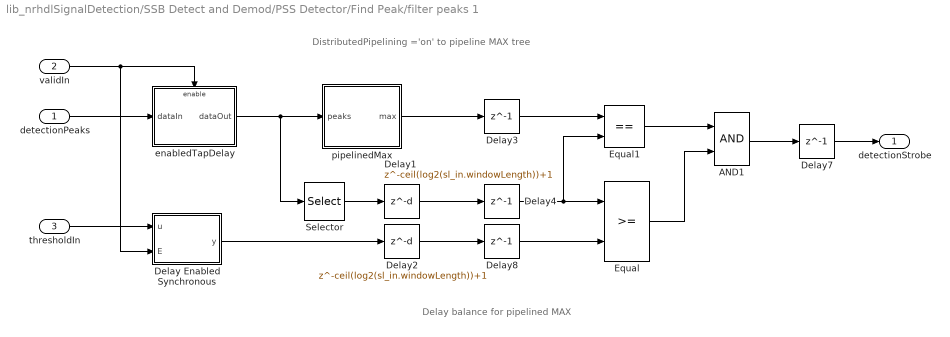
== system lib_nrhdlSignalDetection/SSB Detect and Demod/PSS Detector/Find Peak/filter peaks 1 ==
  note: DistributedPipelining ='on' to pipeline MAX tree
  note: Delay balance for pipelined MAX
  detectionPeaks : Inport
  validIn : Inport  Port=2
  thresholdIn : Inport  Port=3
  AND1 : Logic  AllPortsSameDT=off  OutDataTypeStr=boolean
  Delay Enabled Synchronous : Subsystem  mask(Delay Enabled){DelayLength=ceil(sl_in.windowLength/2), InitialCondition=0.0}
      mask prompts: DelayLength "Simulink:blkprm_prompts:DelayBlkDelayLength"; InitialCondition "Simulink:blkprm_prompts:DelayBlkInitCond"
      mask help: Implements a delay with synchronous enable.
      mask TypeOptions DelayLength: Synchronous Delay/Delay/DelayLength
      mask TypeOptions InitialCondition: Synchronous Delay/Delay/InitialCondition
      mask DialogControl DelayLength Prompt: Delay length:
      mask DialogControl InitialCondition Prompt: Initial condition:
      mask Display:
      | port_label('input', 1, 'u');
      | port_label('input', 2, 'E');
      | text(0.45,0.45, 'Z');
      | DelayLengthStr = get_param(gcbh,'DelayLength');
      | try
      |     DelayLength = eval(DelayLengthStr);
      |     text(0.55,0.55, sprintf('-%d',DelayLength));
      | catch ME
      |     text(0.55,0.55, '-N');
      | end
  Delay1 : Delay  DelayLength=ceil(log2(sl_in.windowLength))+1
  Delay2 : Delay  DelayLength=ceil(log2(sl_in.windowLength))+1
  Delay3 : Delay  DelayLength=1
  Delay4 : Delay  DelayLength=1
  Delay7 : Delay  DelayLength=1
  Delay8 : Delay  DelayLength=1  InitialCondition=1
  Equal : RelationalOperator  OutDataTypeStr=boolean  RndMeth=Simplest  InputSameDT=off
  Equal1 : RelationalOperator  Operator===  OutDataTypeStr=boolean  RndMeth=Simplest  InputSameDT=off
  Selector : Selector  InputPortWidth=sl_in.windowLength  IndexOptions=Index vector (dialog)  Indices=ceil(sl_in.windowLength/2)  OutputSizes=1
  enabledTapDelay : Subsystem
  pipelinedMax : Subsystem
  detectionStrobe : Outport
  wires:
  Delay2/1 -> Delay8/1
  Delay1/1 -> Delay4/1
  pipelinedMax/1(max) -> Delay3/1
  detectionPeaks/1 -> enabledTapDelay/1(dataIn)
  enabledTapDelay/1(dataOut) -> pipelinedMax/1(peaks), Selector/1
  Delay Enabled Synchronous/1(y) -> Delay2/1
  validIn/1 -> enabledTapDelay/Enable, Delay Enabled Synchronous/2(E)
  thresholdIn/1 -> Delay Enabled Synchronous/1(u)
  Delay7/1 -> detectionStrobe/1
  Delay8/1 -> Equal/2
  Selector/1 -> Delay1/1
  AND1/1 -> Delay7/1
  Equal/1 -> AND1/2
  Delay3/1 -> Equal1/1
  Delay4/1 -> Equal/1, Equal1/2
  Equal1/1 -> AND1/1

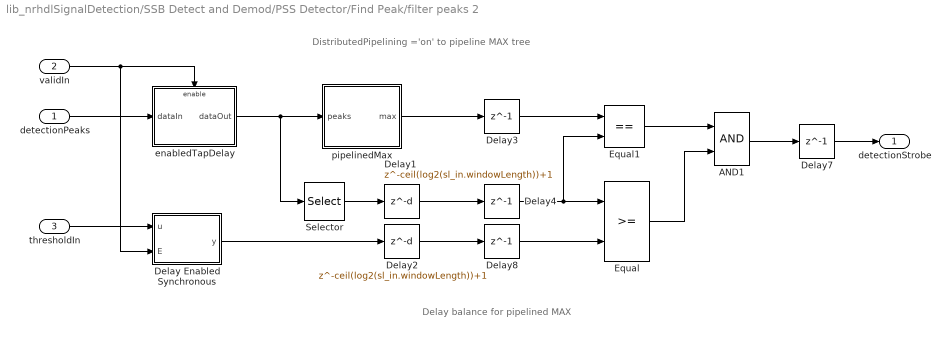
== system lib_nrhdlSignalDetection/SSB Detect and Demod/PSS Detector/Find Peak/filter peaks 2 ==
  note: Delay balance for pipelined MAX
  note: DistributedPipelining ='on' to pipeline MAX tree
  detectionPeaks : Inport
  validIn : Inport  Port=2
  thresholdIn : Inport  Port=3
  AND1 : Logic  AllPortsSameDT=off  OutDataTypeStr=boolean
  Delay Enabled Synchronous : Subsystem  mask(Delay Enabled){DelayLength=ceil(sl_in.windowLength/2), InitialCondition=0.0}
      mask prompts: DelayLength "Simulink:blkprm_prompts:DelayBlkDelayLength"; InitialCondition "Simulink:blkprm_prompts:DelayBlkInitCond"
      mask help: Implements a delay with synchronous enable.
      mask TypeOptions DelayLength: Synchronous Delay/Delay/DelayLength
      mask TypeOptions InitialCondition: Synchronous Delay/Delay/InitialCondition
      mask DialogControl DelayLength Prompt: Delay length:
      mask DialogControl InitialCondition Prompt: Initial condition:
      mask Display:
      | port_label('input', 1, 'u');
      | port_label('input', 2, 'E');
      | text(0.45,0.45, 'Z');
      | DelayLengthStr = get_param(gcbh,'DelayLength');
      | try
      |     DelayLength = eval(DelayLengthStr);
      |     text(0.55,0.55, sprintf('-%d',DelayLength));
      | catch ME
      |     text(0.55,0.55, '-N');
      | end
  Delay1 : Delay  DelayLength=ceil(log2(sl_in.windowLength))+1
  Delay2 : Delay  DelayLength=ceil(log2(sl_in.windowLength))+1
  Delay3 : Delay  DelayLength=1
  Delay4 : Delay  DelayLength=1
  Delay7 : Delay  DelayLength=1
  Delay8 : Delay  DelayLength=1  InitialCondition=1
  Equal : RelationalOperator  OutDataTypeStr=boolean  RndMeth=Simplest  InputSameDT=off
  Equal1 : RelationalOperator  Operator===  OutDataTypeStr=boolean  RndMeth=Simplest  InputSameDT=off
  Selector : Selector  InputPortWidth=sl_in.windowLength  IndexOptions=Index vector (dialog)  Indices=ceil(sl_in.windowLength/2)  OutputSizes=1
  enabledTapDelay : Subsystem
  pipelinedMax : Subsystem
  detectionStrobe : Outport
  wires:
  Equal1/1 -> AND1/1
  Delay4/1 -> Equal1/2, Equal/1
  Delay3/1 -> Equal1/1
  Equal/1 -> AND1/2
  AND1/1 -> Delay7/1
  Selector/1 -> Delay1/1
  Delay8/1 -> Equal/2
  Delay7/1 -> detectionStrobe/1
  thresholdIn/1 -> Delay Enabled Synchronous/1(u)
  validIn/1 -> Delay Enabled Synchronous/2(E), enabledTapDelay/Enable
  Delay Enabled Synchronous/1(y) -> Delay2/1
  enabledTapDelay/1(dataOut) -> Selector/1, pipelinedMax/1(peaks)
  detectionPeaks/1 -> enabledTapDelay/1(dataIn)
  pipelinedMax/1(max) -> Delay3/1
  Delay1/1 -> Delay4/1
  Delay2/1 -> Delay8/1

== system lib_nrhdlSignalDetection/SSB Detect and Demod/PSS Detector/signalMagAverage/Synchronous Enabled Nfft Sample Delay  ==
  dataIn : Inport
  en : Inport  Port=2
  Delay1 : Delay  DelayLength=sl_in.Nfft  InitialCondition=0  ShowEnablePort=on
      settings: InputPortMap=u0,e6
  State Control : StateControl  StateControl=Synchronous
  dataOut : Outport  VectorParamsAs1DForOutWhenUnconnected=off
  wires:
  en/1 -> Delay1/2
  dataIn/1 -> Delay1/1
  Delay1/1 -> dataOut/1

== system lib_nrhdlSignalDetection/SSB Detect and Demod/PSS Detector/Find Peak/Delay Enabled Synchronous/Synchronous Delay ==
  u : Inport
  E : Inport  Port=2
  Delay : Delay  DelayLength=DelayLength  InitialCondition=InitialCondition  ShowEnablePort=on
      settings: InputPortMap=u0,e6
  State Control : StateControl  StateControl=Synchronous
  y : Outport
  wires:
  u/1 -> Delay/1
  E/1 -> Delay/2
  Delay/1 -> y/1

== system lib_nrhdlSignalDetection/SSB Detect and Demod/PSS Detector/Find Peak/filter peaks 0/Delay Enabled Synchronous ==
  u : Inport
  E : Inport  Port=2
  Synchronous Delay : Subsystem
  y : Outport
  wires:
  Synchronous Delay/1(y) -> y/1
  E/1 -> Synchronous Delay/2(E)
  u/1 -> Synchronous Delay/1(u)

== system lib_nrhdlSignalDetection/SSB Detect and Demod/PSS Detector/Find Peak/filter peaks 0/enabledTapDelay ==
  dataIn : Inport
  Enable : EnablePort
  State Control : StateControl  StateControl=Synchronous
  Tapped Delay : simulink/Discrete/Tapped Delay  vinit=0.0  samptime=-1  NumDelays=sl_in.windowLength  DelayOrder=Oldest  includeCurrent=off
  dataOut : Outport
  wires:
  Tapped Delay/1 -> dataOut/1
  dataIn/1 -> Tapped Delay/1

== system lib_nrhdlSignalDetection/SSB Detect and Demod/PSS Detector/Find Peak/filter peaks 0/pipelinedMax ==
  peaks : Inport
  Delay1 : Delay  DelayLength=ceil(log2(sl_in.windowLength))+1
  Max : MinMax  Function=max
  max : Outport
  wires:
  Max/1 -> Delay1/1
  Delay1/1 -> max/1
  peaks/1 -> Max/1

== system lib_nrhdlSignalDetection/SSB Detect and Demod/PSS Detector/Find Peak/filter peaks 1/Delay Enabled Synchronous ==
  u : Inport
  E : Inport  Port=2
  Synchronous Delay : Subsystem
  y : Outport
  wires:
  u/1 -> Synchronous Delay/1(u)
  E/1 -> Synchronous Delay/2(E)
  Synchronous Delay/1(y) -> y/1

== system lib_nrhdlSignalDetection/SSB Detect and Demod/PSS Detector/Find Peak/filter peaks 1/enabledTapDelay ==
  dataIn : Inport
  Enable : EnablePort
  State Control : StateControl  StateControl=Synchronous
  Tapped Delay : simulink/Discrete/Tapped Delay  vinit=0.0  samptime=-1  NumDelays=sl_in.windowLength  DelayOrder=Oldest  includeCurrent=off
  dataOut : Outport
  wires:
  dataIn/1 -> Tapped Delay/1
  Tapped Delay/1 -> dataOut/1

== system lib_nrhdlSignalDetection/SSB Detect and Demod/PSS Detector/Find Peak/filter peaks 1/pipelinedMax ==
  peaks : Inport
  Delay1 : Delay  DelayLength=ceil(log2(sl_in.windowLength))+1
  Max : MinMax  Function=max
  max : Outport
  wires:
  peaks/1 -> Max/1
  Delay1/1 -> max/1
  Max/1 -> Delay1/1

== system lib_nrhdlSignalDetection/SSB Detect and Demod/PSS Detector/Find Peak/filter peaks 2/Delay Enabled Synchronous ==
  u : Inport
  E : Inport  Port=2
  Synchronous Delay : Subsystem
  y : Outport
  wires:
  Synchronous Delay/1(y) -> y/1
  E/1 -> Synchronous Delay/2(E)
  u/1 -> Synchronous Delay/1(u)

== system lib_nrhdlSignalDetection/SSB Detect and Demod/PSS Detector/Find Peak/filter peaks 2/enabledTapDelay ==
  dataIn : Inport
  Enable : EnablePort
  State Control : StateControl  StateControl=Synchronous
  Tapped Delay : simulink/Discrete/Tapped Delay  vinit=0.0  samptime=-1  NumDelays=sl_in.windowLength  DelayOrder=Oldest  includeCurrent=off
  dataOut : Outport
  wires:
  Tapped Delay/1 -> dataOut/1
  dataIn/1 -> Tapped Delay/1

== system lib_nrhdlSignalDetection/SSB Detect and Demod/PSS Detector/Find Peak/filter peaks 2/pipelinedMax ==
  peaks : Inport
  Delay1 : Delay  DelayLength=ceil(log2(sl_in.windowLength))+1
  Max : MinMax  Function=max
  max : Outport
  wires:
  Max/1 -> Delay1/1
  Delay1/1 -> max/1
  peaks/1 -> Max/1

== system lib_nrhdlSignalDetection/SSB Detect and Demod/PSS Detector/Find Peak/filter peaks 0/Delay Enabled Synchronous/Synchronous Delay ==
  u : Inport
  E : Inport  Port=2
  Delay : Delay  DelayLength=DelayLength  InitialCondition=InitialCondition  ShowEnablePort=on
      settings: InputPortMap=u0,e6
  State Control : StateControl  StateControl=Synchronous
  y : Outport
  wires:
  u/1 -> Delay/1
  E/1 -> Delay/2
  Delay/1 -> y/1

== system lib_nrhdlSignalDetection/SSB Detect and Demod/PSS Detector/Find Peak/filter peaks 1/Delay Enabled Synchronous/Synchronous Delay ==
  u : Inport
  E : Inport  Port=2
  Delay : Delay  DelayLength=DelayLength  InitialCondition=InitialCondition  ShowEnablePort=on
      settings: InputPortMap=u0,e6
  State Control : StateControl  StateControl=Synchronous
  y : Outport
  wires:
  Delay/1 -> y/1
  E/1 -> Delay/2
  u/1 -> Delay/1

== system lib_nrhdlSignalDetection/SSB Detect and Demod/PSS Detector/Find Peak/filter peaks 2/Delay Enabled Synchronous/Synchronous Delay ==
  u : Inport
  E : Inport  Port=2
  Delay : Delay  DelayLength=DelayLength  InitialCondition=InitialCondition  ShowEnablePort=on
      settings: InputPortMap=u0,e6
  State Control : StateControl  StateControl=Synchronous
  y : Outport
  wires:
  u/1 -> Delay/1
  E/1 -> Delay/2
  Delay/1 -> y/1

== matlab function lib_nrhdlSignalDetection/SSB Detect and Demod/PSS Detector/Find Peak/register PSS ID ==
  data: A input; selectedPSS output; B input; C input; valid output; validIn input; start input
function [selectedPSS, valid] = registerPSSID(A, B, C, validIn, start)

persistent started pss_reg pss_valid

if isempty(pss_reg)
    started = false;
    pss_reg = fi(0,0,2,0);
    pss_valid = false;
end

valid = pss_valid;
selectedPSS = pss_reg;

if start
    started(:) = 1;
    pss_valid(:) = 0;
    pss_reg(:) = 0;
end

if started
    if validIn && ~pss_valid
        if(A||B||C)
            pss_valid(:) = true;
        
            if A == 1
                pss_reg(:) = 0;
            elseif B == 1
                pss_reg(:) = 1;
            else
                pss_reg(:) = 2;
            end
        end
    end
end

== matlab function lib_nrhdlSignalDetection/SSB Detect and Demod/PSS Detector/Stream Synchronizer/MATLAB Function ==
  data: wrAddr output; wrEn output; rdAddr output; pop input; push input; validOut output; depth parameter
function [wrAddr,wrEn,rdAddr, validOut] = ofdmDataSync(pop,push,depth)
    %#codegen
    
    coder.extrinsic('warning');
    coder.extrinsic('num2str');
    
    persistent reg level;
    
    %------------------------------------------------------------------------
    % Constants
    %------------------------------------------------------------------------
    
    addrWL = nextpow2(depth);
    
    %------------------------------------------------------------------------
    % Persistent variable initialization
    %------------------------------------------------------------------------
    
    if isempty(reg)
        
        reg = struct(...
            'wrAddr',       fi(0,0,addrWL,0,hdlfimath), ...
            'rdAddr',       fi(0,0,addrWL,0,hdlfimath), ...
            'valid',        false);
        
        % For generating warnings during simulation only.
        level = int16(0);
        
    end
    
    %------------------------------------------------------------------------
    % Outputs
    %------------------------------------------------------------------------
    
    wrAddr   = reg.wrAddr;
    wrEn     = push;
    rdAddr   = reg.rdAddr;
    validOut = reg.valid;
    
    %------------------------------------------------------------------------
    % Calculate next state values
    %------------------------------------------------------------------------
    
    % Initialize next state
    next = reg;
    
    if pop
        next.rdAddr(:)  = reg.rdAddr + 1;
        level(:)        = level - 1;
        
        if level < 0
            warning('Buffer underflow: attempt to pop data out of empty buffer.');
        end
    end
    
    if push
        next.wrAddr(:)     = reg.wrAddr+1;
        level(:)      = level+1;
        
        if level > depth            
            warning(['Buffer overflow: attempt to push data into full buffer. Level = ', num2str(level), '.']);
        end
        
    end
    
    next.valid = pop; 
    
    % Update state    
    reg = next;
end

== matlab function lib_nrhdlSignalDetection/SSB Detect and Demod/Stream Synchronizer/MATLAB Function ==
  data: wrAddr output; wrEn output; rdAddr output; pop input; push input; validOut output; depth parameter
function [wrAddr,wrEn,rdAddr, validOut] = ofdmDataSync(pop,push,depth)
    %#codegen
    
    coder.extrinsic('warning');
    coder.extrinsic('num2str');
    
    persistent reg level;
    
    %------------------------------------------------------------------------
    % Constants
    %------------------------------------------------------------------------
    
    addrWL = nextpow2(depth);
    
    %------------------------------------------------------------------------
    % Persistent variable initialization
    %------------------------------------------------------------------------
    
    if isempty(reg)
        
        reg = struct(...
            'wrAddr',       fi(0,0,addrWL,0,hdlfimath), ...
            'rdAddr',       fi(0,0,addrWL,0,hdlfimath), ...
            'valid',        false);
        
        % For generating warnings during simulation only.
        level = int16(0);
        
    end
    
    %------------------------------------------------------------------------
    % Outputs
    %------------------------------------------------------------------------
    
    wrAddr   = reg.wrAddr;
    wrEn     = push;
    rdAddr   = reg.rdAddr;
    validOut = reg.valid;
    
    %------------------------------------------------------------------------
    % Calculate next state values
    %------------------------------------------------------------------------
    
    % Initialize next state
    next = reg;
    
    if pop
        next.rdAddr(:)  = reg.rdAddr + 1;
        level(:)        = level - 1;
        
        if level < 0
            warning('Buffer underflow: attempt to pop data out of empty buffer.');
        end
    end
    
    if push
        next.wrAddr(:)     = reg.wrAddr+1;
        level(:)      = level+1;
        
        if level > depth            
            warning(['Buffer overflow: attempt to push data into full buffer. Level = ', num2str(level), '.']);
        end
        
    end
    
    next.valid = pop; 
    
    % Update state    
    reg = next;
end

== matlab function lib_nrhdlSignalDetection/SSB Detect and Demod/scsSelection/Transient Removal ==
  data: dataIn input; dataOut output; validIn input; validOut output; TransientLength parameter
function [dataOut, validOut] = removeTransient(dataIn, validIn, TransientLength)
%#codegen

persistent count dataOutReg validOutReg;

if isempty(count)
    count = fi(0,0,nextpow2(TransientLength+1),0,hdlfimath);
    dataOutReg = cast(0,'like',dataIn);
    validOutReg = false;
end

dataOut  = dataOutReg;
validOut = validOutReg;

if validIn && (count == TransientLength)
    dataOutReg(:) = dataIn;
    validOutReg(:) = true;
else
    dataOutReg(:) = dataOutReg;
    validOutReg(:) = false;
end

if validIn && count ~= TransientLength
    count(:) = count + 1;
end

== matlab function lib_nrhdlSignalDetection/SSB Detect and Demod/OFDM Demodulator/OFDM Demod Controller ==
  data: validIn input; startIn input; validOut output; done output
function [validOut, done] = ofdmDemodController(validIn, startIn)
    
    persistent reg
    
    Nfft = 256;
    Ncp = 18;
    numOFDMSymbols = 4;
    samplesPerOFDMSymbol = Nfft + Ncp;
    ofdmCountWL = nextpow2(samplesPerOFDMSymbol*numOFDMSymbols);
    
    if isempty(reg)
        reg = struct(...
            'valid', false, ...
            'started', false,...
            'done', false,...
            'ofdmCount', fi(0,0,ofdmCountWL,0)...
            );
    end
    
    validOut = reg.valid;
    done = reg.done;
    
    next = reg;

    if reg.done
        next.done(:) = false;
    end
        
    if startIn && validIn
        next.valid(:) = 1;
        next.started(:) = 1;
        next.ofdmCount(:) = 0;
    elseif validIn && reg.started
        next.valid(:) = 1;
        if reg.ofdmCount == samplesPerOFDMSymbol*numOFDMSymbols-2
            next.started(:) = 0;
            next.ofdmCount(:) = 0;
            next.done(:) = true;
        else
            next.ofdmCount(:) = reg.ofdmCount + 1;
        end
    else
        next.valid(:) = 0;
    end
    
    reg = next;
    
end
